simulink model "FeedForwardCascadare"  (R2024b)
settings: Solver=VariableStepAuto  StartTime=0.0  StopTime=600  RelTol=1e-3
values from neighbouring files (symbols this model uses):
  A = 332.5    [scriptProiect.m]
  C = 9    [scriptProiect.m]
  h0 = 10.5    [scriptProiect.m]
  k = 0.035    [scriptProiect.m]
  k1 = 0.624    [scriptProiect.m]
  k2 = -0.015    [scriptProiect.m]
  k3 = -0.0006    [scriptProiect.m]
  keta = 8 * 10^-5    (= 8e-05)    [scriptProiect.m]
  Kr1 = Tp1 / Kf1 / T01    (= 0.286274509804)    [scriptProiect.m]
  Kr2 = Tf2 / Kf2 / T02    (= 40)    [scriptProiect.m]
  q0 = 29.2    [scriptProiect.m]
  Rm = 3    [scriptProiect.m]
  Ti1 = Tp1    (= 0.73)    [scriptProiect.m]
  Ti2 = Tf2    (= 260)    [scriptProiect.m]
libraries: slpidlib x2
settings Model: Creator=Teo  LastModifiedBy=Teo

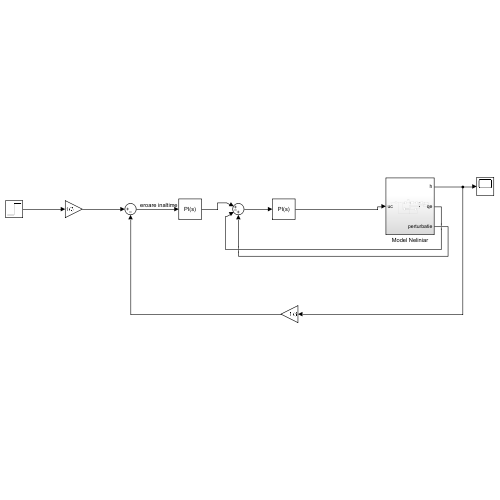
[thumbnail: Simulink's stored preview of the top-level diagram]
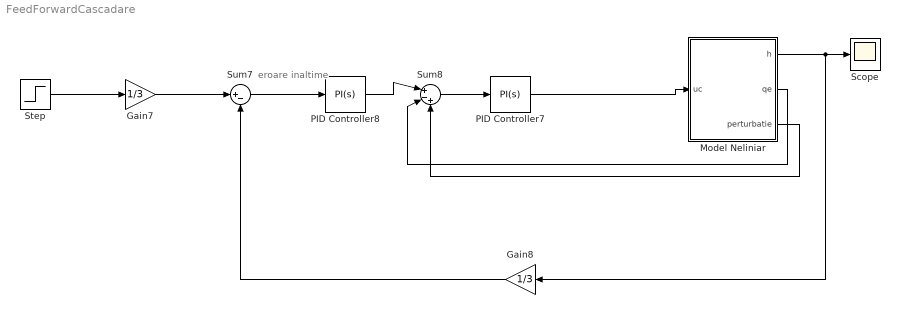
== system FeedForwardCascadare ==
  note: eroare inaltime
  Gain7 : Gain  Gain=1/3
  Gain8 : Gain  Gain=1/3
  Model Neliniar : Subsystem
  PID Controller7 : slpidlib/PID Controller  Controller=PI  Form=Parallel  TimeDomain=Continuous-time  UseExternalTs=off  SampleTime=-1  IntegratorMethod=Forward Euler  FilterMethod=Forward Euler  ControllerParametersSource=internal  P=Kr1  I=Kr1/Ti1  UseKiTs=off  D=0  UseExternalDerivativeSource=off  N=100  UseFilter=on  TunerSelectOption=Transfer Function Based (PID Tuner App)  InitialConditionSource=internal  InitialConditionForIntegrator=u0  InitialConditionForFilter=0  DifferentiatorICPrevScaledInput=0  ExternalReset=none  TrackingMode=off  Kt=1  LimitOutput=off  SatLimitsSource=internal  UpperSaturationLimit=inf  LowerSaturationLimit=-inf  LinearizeAsGain=on  AntiWindupMode=none  Kb=1  LimitIntegrator=off  UpperIntegratorSaturationLimit=inf  LowerIntegratorSaturationLimit=-inf  POutMin=[]  POutMax=[]  IOutMin=[]  IOutMax=[]  DOutMin=[]  DOutMax=[]  NOutMin=[]  NOutMax=[]  SumOutMin=[]  SumOutMax=[]  SaturationOutMin=[]  SaturationOutMax=[]  PParamMin=[]  PParamMax=[]  IParamMin=[]  IParamMax=[]  DParamMin=[]  DParamMax=[]  NParamMin=[]  NParamMax=[]  KbParamMin=[]  KbParamMax=[]  KtParamMin=[]  KtParamMax=[]  KbOutMin=[]  KbOutMax=[]  KtOutMin=[]  KtOutMax=[]  IntegratorOutMin=[]  IntegratorOutMax=[]  FilterOutMin=[]  FilterOutMax=[]  SumI1OutMin=[]  SumI1OutMax=[]  SumI2OutMin=[]  SumI2OutMax=[]  SumI3OutMin=[]  SumI3OutMax=[]  SumI4OutMin=[]  SumI4OutMax=[]  SumDOutMin=[]  SumDOutMax=[]  DifferentiatorOutMin=[]  DifferentiatorOutMax=[]  FilterDiffOutCoefMin=[]  FilterDiffOutCoefMax=[]  ReciprocalOutMin=[]  ReciprocalOutMax=[]  SumDenOutMin=[]  SumDenOutMax=[]  SumNumOutMin=[]  SumNumOutMax=[]  DivideOutMin=[]  DivideOutMax=[]  UdiffTsProdOutMin=[]  UdiffTsProdOutMax=[]  NTsProdOutMin=[]  NTsProdOutMax=[]  UintegralTsProdOutMin=[]  UintegralTsProdOutMax=[]  UngainTsProdOutMin=[]  UngainTsProdOutMax=[]  ClampingZeroOutDataTypeStr=Inherit: Inherit via back propagation  ClampingZeroOutMin=[]  ClampingZeroOutMax=[]  FilterDenConstantOutDataTypeStr=Inherit: Inherit via back propagation  FilterDenConstantOutMin=[]  FilterDenConstantOutMax=[]  PCopyOutDataTypeStr=Inherit: Inherit via back propagation  PCopyOutMin=[]  PCopyOutMax=[]  NCopyOutDataTypeStr=Inherit: Inherit via back propagation  NCopyOutMin=[]  NCopyOutMax=[]  IntegratorContinuousStateAttributes=''  IntegratorStateMustResolveToSignalObject=off  IntegratorRTWStateStorageClass=Auto  FilterContinuousStateAttributes=''  FilterStateMustResolveToSignalObject=off  FilterRTWStateStorageClass=Auto  ParallelPVariant=InternalParameters  IdealPVariant=Disabled  IVariant=InternalParameters  DVariant=Disabled  IntegratorVariant=Continuous  SatVariant=Disabled  AWVariant=Passthrough  PCopyVariant=Disabled  TRVariant=Disabled  FdbkBlocksVariant=Forward  IdealPFdbkVariant=Disabled  SatFdbkVariant=Disabled  DerivativeFilterVariant=Disabled  NVariant=Disabled  NCopyVariant=Disabled_SignalSpec  FilterICVariant=Disabled  IntegratorICVariant=InternalICs  ExternalResetVariant=Disabled  TRSumVariant=Passthrough  SumFdbkVariant=Disabled  SumVariant=Sum_PI  TsampFilterVariant=InternalTs  TsampNgainVariant=Passthrough  TsampIntegralVariant=Disabled_SignalSpec  ExternalSaturationOutDataTypeStr=Inherit: Same as second input  DerivativeSourceVariant=Disabled  PreIntVariant=InternalPreInt
  PID Controller8 : slpidlib/PID Controller  Controller=PI  Form=Parallel  TimeDomain=Continuous-time  UseExternalTs=off  SampleTime=-1  IntegratorMethod=Forward Euler  FilterMethod=Forward Euler  ControllerParametersSource=internal  P=Kr2  I=Kr2/Ti2  UseKiTs=off  D=0  UseExternalDerivativeSource=off  N=100  UseFilter=on  TunerSelectOption=Transfer Function Based (PID Tuner App)  InitialConditionSource=internal  InitialConditionForIntegrator=q0  InitialConditionForFilter=0  DifferentiatorICPrevScaledInput=0  ExternalReset=none  TrackingMode=off  Kt=1  LimitOutput=off  SatLimitsSource=internal  UpperSaturationLimit=inf  LowerSaturationLimit=-inf  LinearizeAsGain=on  AntiWindupMode=none  Kb=1  LimitIntegrator=off  UpperIntegratorSaturationLimit=inf  LowerIntegratorSaturationLimit=-inf  POutMin=[]  POutMax=[]  IOutMin=[]  IOutMax=[]  DOutMin=[]  DOutMax=[]  NOutMin=[]  NOutMax=[]  SumOutMin=[]  SumOutMax=[]  SaturationOutMin=[]  SaturationOutMax=[]  PParamMin=[]  PParamMax=[]  IParamMin=[]  IParamMax=[]  DParamMin=[]  DParamMax=[]  NParamMin=[]  NParamMax=[]  KbParamMin=[]  KbParamMax=[]  KtParamMin=[]  KtParamMax=[]  KbOutMin=[]  KbOutMax=[]  KtOutMin=[]  KtOutMax=[]  IntegratorOutMin=[]  IntegratorOutMax=[]  FilterOutMin=[]  FilterOutMax=[]  SumI1OutMin=[]  SumI1OutMax=[]  SumI2OutMin=[]  SumI2OutMax=[]  SumI3OutMin=[]  SumI3OutMax=[]  SumI4OutMin=[]  SumI4OutMax=[]  SumDOutMin=[]  SumDOutMax=[]  DifferentiatorOutMin=[]  DifferentiatorOutMax=[]  FilterDiffOutCoefMin=[]  FilterDiffOutCoefMax=[]  ReciprocalOutMin=[]  ReciprocalOutMax=[]  SumDenOutMin=[]  SumDenOutMax=[]  SumNumOutMin=[]  SumNumOutMax=[]  DivideOutMin=[]  DivideOutMax=[]  UdiffTsProdOutMin=[]  UdiffTsProdOutMax=[]  NTsProdOutMin=[]  NTsProdOutMax=[]  UintegralTsProdOutMin=[]  UintegralTsProdOutMax=[]  UngainTsProdOutMin=[]  UngainTsProdOutMax=[]  ClampingZeroOutDataTypeStr=Inherit: Inherit via back propagation  ClampingZeroOutMin=[]  ClampingZeroOutMax=[]  FilterDenConstantOutDataTypeStr=Inherit: Inherit via back propagation  FilterDenConstantOutMin=[]  FilterDenConstantOutMax=[]  PCopyOutDataTypeStr=Inherit: Inherit via back propagation  PCopyOutMin=[]  PCopyOutMax=[]  NCopyOutDataTypeStr=Inherit: Inherit via back propagation  NCopyOutMin=[]  NCopyOutMax=[]  IntegratorContinuousStateAttributes=''  IntegratorStateMustResolveToSignalObject=off  IntegratorRTWStateStorageClass=Auto  FilterContinuousStateAttributes=''  FilterStateMustResolveToSignalObject=off  FilterRTWStateStorageClass=Auto  ParallelPVariant=InternalParameters  IdealPVariant=Disabled  IVariant=InternalParameters  DVariant=Disabled  IntegratorVariant=Continuous  SatVariant=Disabled  AWVariant=Passthrough  PCopyVariant=Disabled  TRVariant=Disabled  FdbkBlocksVariant=Forward  IdealPFdbkVariant=Disabled  SatFdbkVariant=Disabled  DerivativeFilterVariant=Disabled  NVariant=Disabled  NCopyVariant=Disabled_SignalSpec  FilterICVariant=Disabled  IntegratorICVariant=InternalICs  ExternalResetVariant=Disabled  TRSumVariant=Passthrough  SumFdbkVariant=Disabled  SumVariant=Sum_PI  TsampFilterVariant=InternalTs  TsampNgainVariant=Passthrough  TsampIntegralVariant=Disabled_SignalSpec  ExternalSaturationOutDataTypeStr=Inherit: Same as second input  DerivativeSourceVariant=Disabled  PreIntVariant=InternalPreInt
  Scope : Scope
  Step : Step  Time=0  After=13  SampleTime=0
  Sum7 : Sum  Inputs=|+-
  Sum8 : Sum  Inputs=|+-+
  wires:
  Step/1 -> Gain7/1
  Sum7/1 -> PID Controller8/1
  PID Controller7/1 -> Model Neliniar/1(uc)
  Gain7/1 -> Sum7/1
  Gain8/1 -> Sum7/2
  PID Controller8/1 -> Sum8/1
  Model Neliniar/3(perturbatie) -> Sum8/3
  Model Neliniar/2(qe) -> Sum8/2
  Model Neliniar/1(h) -> Gain8/1, Scope/1
  Sum8/1 -> PID Controller7/1

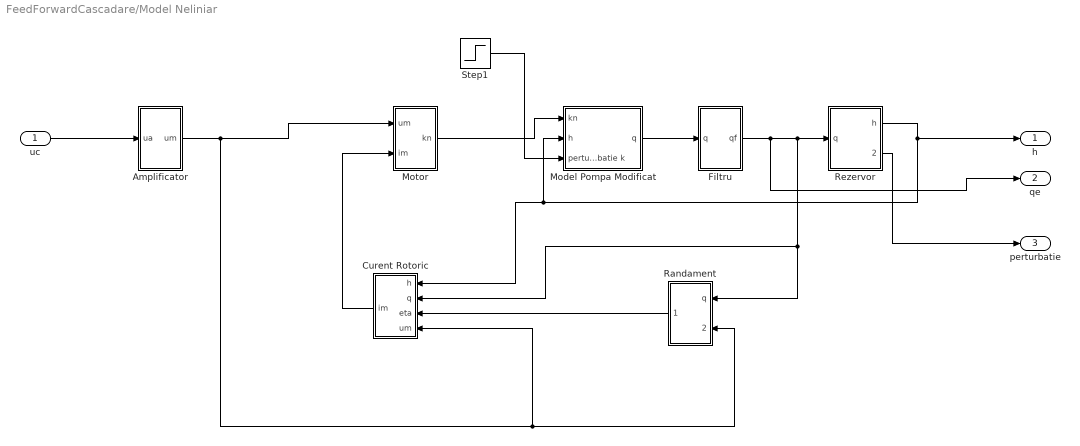
== system FeedForwardCascadare/Model Neliniar ==
  uc : Inport
  Amplificator : Subsystem
  Curent Rotoric : Subsystem
  Filtru : Subsystem
  Model Pompa Modificat : Subsystem
  Motor : Subsystem
  "Randament " : Subsystem
  Rezervor : Subsystem
  Step1 : Step  Time=300  After=0.5*k  SampleTime=0
  h : Outport
  qe : Outport  Port=2
  perturbatie : Outport  Port=3
  wires:
  Curent Rotoric/1(im) -> Motor/2(im)
  "Randament "/1(eta) -> Curent Rotoric/3(eta)
  Motor/1(kn) -> Model Pompa Modificat/1(kn)
  Rezervor/1(h) -> h/1, Model Pompa Modificat/2(h), Curent Rotoric/1(h)
  Filtru/1(qf) -> qe/1, "Randament "/1(q), Curent Rotoric/2(q), Rezervor/1(q)
  Model Pompa Modificat/1(q) -> Filtru/1(q)
  uc/1 -> Amplificator/1(ua)
  Amplificator/1(um) -> "Randament "/2(um), Curent Rotoric/4(um), Motor/1(um)
  Rezervor/2(perturbatie) -> perturbatie/1
  Step1/1 -> Model Pompa Modificat/3(perturbatie k)

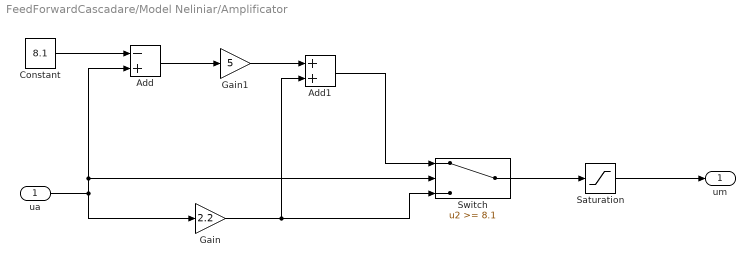
== system FeedForwardCascadare/Model Neliniar/Amplificator ==
  ua : Inport
  Add : Sum  Inputs=-+
  Add1 : Sum
  Constant : Constant  Value=8.1
  Gain : Gain  Gain=2.2
  Gain1 : Gain  Gain=5
  Saturation : Saturate  UpperLimit=22  LowerLimit=0
  Switch : Switch  Threshold=8.1  SaturateOnIntegerOverflow=off  InputSameDT=off
  um : Outport
  wires:
  Add/1 -> Gain1/1
  Add1/1 -> Switch/1
  Switch/1 -> Saturation/1
  Constant/1 -> Add/1
  Saturation/1 -> um/1
  Gain/1 -> Switch/3, Add1/2
  ua/1 -> Add/2, Switch/2, Gain/1
  Gain1/1 -> Add1/1

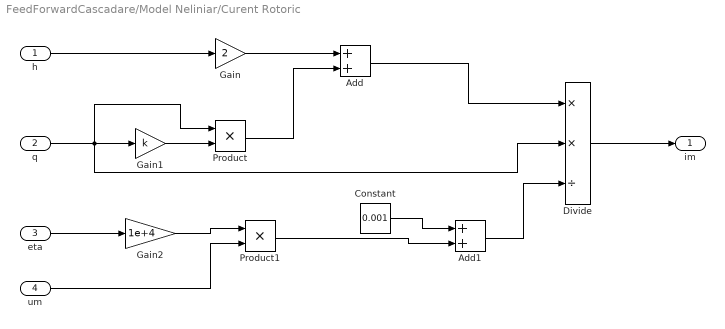
== system FeedForwardCascadare/Model Neliniar/Curent Rotoric ==
  h : Inport
  q : Inport  Port=2
  eta : Inport  Port=3
  um : Inport  Port=4
  Add : Sum
  Add1 : Sum
  Constant : Constant  Value=0.001
  Divide : Product  Inputs=**/
  Gain : Gain  Gain=2
  Gain1 : Gain  Gain=k
  Gain2 : Gain  Gain=1e+4
  Product : Product
  Product1 : Product
  im : Outport
  wires:
  Gain1/1 -> Product/2
  Gain/1 -> Add/1
  Gain2/1 -> Product1/1
  q/1 -> Divide/2, Product/1, Gain1/1
  Add1/1 -> Divide/3
  Product1/1 -> Add1/2
  um/1 -> Product1/2
  Add/1 -> Divide/1
  Product/1 -> Add/2
  eta/1 -> Gain2/1
  h/1 -> Gain/1
  Constant/1 -> Add1/1
  Divide/1 -> im/1

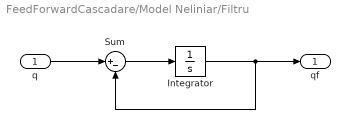
== system FeedForwardCascadare/Model Neliniar/Filtru ==
  q : Inport
  Integrator : Integrator  InitialCondition=q0
  Sum : Sum  Inputs=|+-
  qf : Outport
  wires:
  q/1 -> Sum/1
  Integrator/1 -> qf/1, Sum/2
  Sum/1 -> Integrator/1

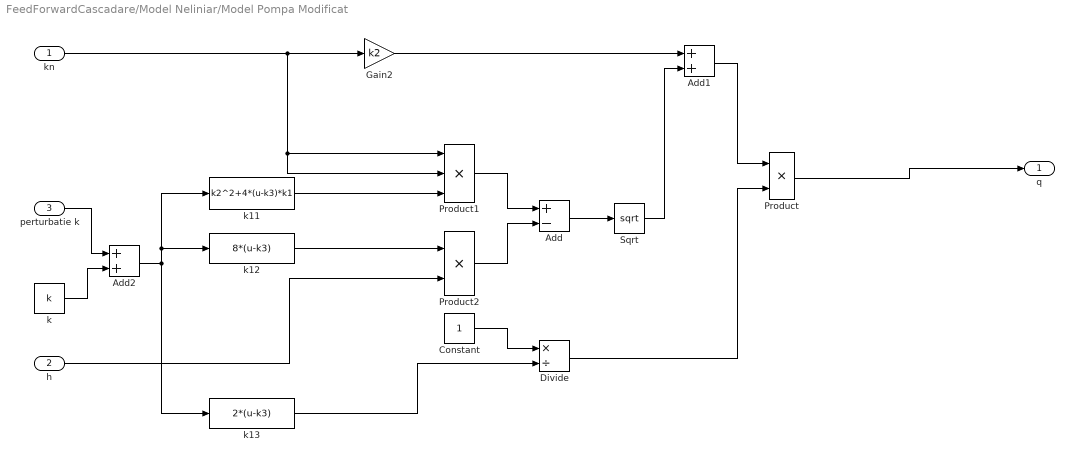
== system FeedForwardCascadare/Model Neliniar/Model Pompa Modificat ==
  kn : Inport
  h : Inport  Port=2
  perturbatie k : Inport  Port=3
  Add : Sum  Inputs=+-
  Add1 : Sum
  Add2 : Sum
  Constant : Constant
  Divide : Product  Inputs=*/
  Gain2 : Gain  Gain=k2
  Product : Product
  Product1 : Product  Inputs=3
  Product2 : Product
  Sqrt : Sqrt
  k : Constant  Value=k
  k11 : Fcn  Expr=k2^2+4*(u-k3)*k1
  k12 : Fcn  Expr=8*(u-k3)
  k13 : Fcn  Expr=2*(u-k3)
  q : Outport
  wires:
  h/1 -> Product2/2
  Sqrt/1 -> Add1/2
  Add1/1 -> Product/1
  Add/1 -> Sqrt/1
  Gain2/1 -> Add1/1
  kn/1 -> Product1/2, Product1/1, Gain2/1
  Product1/1 -> Add/1
  Product2/1 -> Add/2
  perturbatie k/1 -> Add2/1
  k/1 -> Add2/2
  Add2/1 -> k12/1, k11/1, k13/1
  k11/1 -> Product1/3
  k12/1 -> Product2/1
  Constant/1 -> Divide/1
  k13/1 -> Divide/2
  Divide/1 -> Product/2
  Product/1 -> q/1

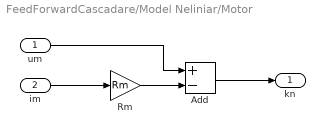
== system FeedForwardCascadare/Model Neliniar/Motor ==
  um : Inport
  im : Inport  Port=2
  Add : Sum  Inputs=+-
  Rm : Gain  Gain=Rm
  kn : Outport
  wires:
  im/1 -> Rm/1
  Rm/1 -> Add/2
  um/1 -> Add/1
  Add/1 -> kn/1

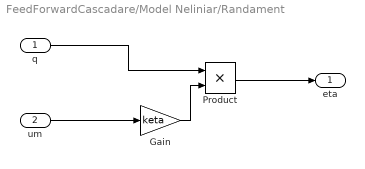
== system FeedForwardCascadare/Model Neliniar/Randament  ==
  q : Inport
  um : Inport  Port=2
  Gain : Gain  Gain=keta
  Product : Product
  eta : Outport
  wires:
  um/1 -> Gain/1
  Product/1 -> eta/1
  Gain/1 -> Product/2
  q/1 -> Product/1

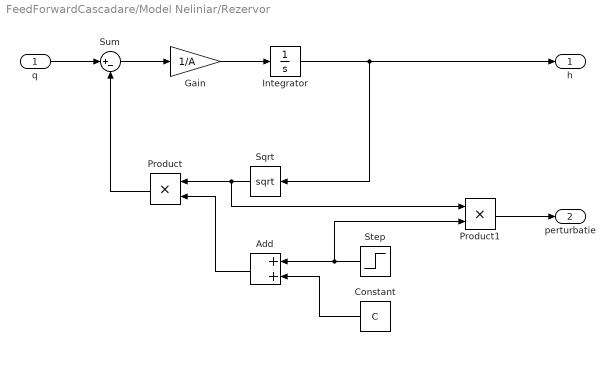
== system FeedForwardCascadare/Model Neliniar/Rezervor ==
  q : Inport
  Add : Sum
  Constant : Constant  Value=C
  Gain : Gain  Gain=1/A
  Integrator : Integrator  InitialCondition=h0
  Product : Product
  Product1 : Product
  Sqrt : Sqrt
  Step : Step  Time=400  After=2  SampleTime=0
  Sum : Sum  Inputs=|+-
  h : Outport
  perturbatie : Outport  Port=2
  wires:
  Gain/1 -> Integrator/1
  Sum/1 -> Gain/1
  Integrator/1 -> Sqrt/1, h/1
  q/1 -> Sum/1
  Product/1 -> Sum/2
  Sqrt/1 -> Product1/1, Product/1
  Add/1 -> Product/2
  Constant/1 -> Add/2
  Step/1 -> Product1/2, Add/1
  Product1/1 -> perturbatie/1
